simulink model "es2"  (R2024b)
settings: Solver=VariableStepAuto  StartTime=0.0  StopTime=30  RelTol=1e-3
undefined symbols (not defined in the file or in its folder): dspblkCoreblockFVToolHelper, gcbh
libraries: vrlib x1
settings Model: Creator=mattia  LastModifiedBy=elima

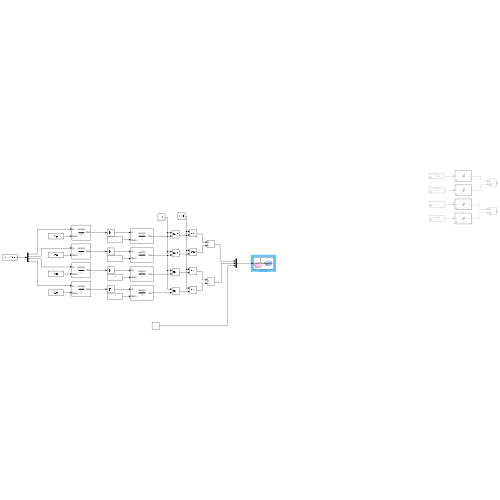
[thumbnail: Simulink's stored preview of the top-level diagram]
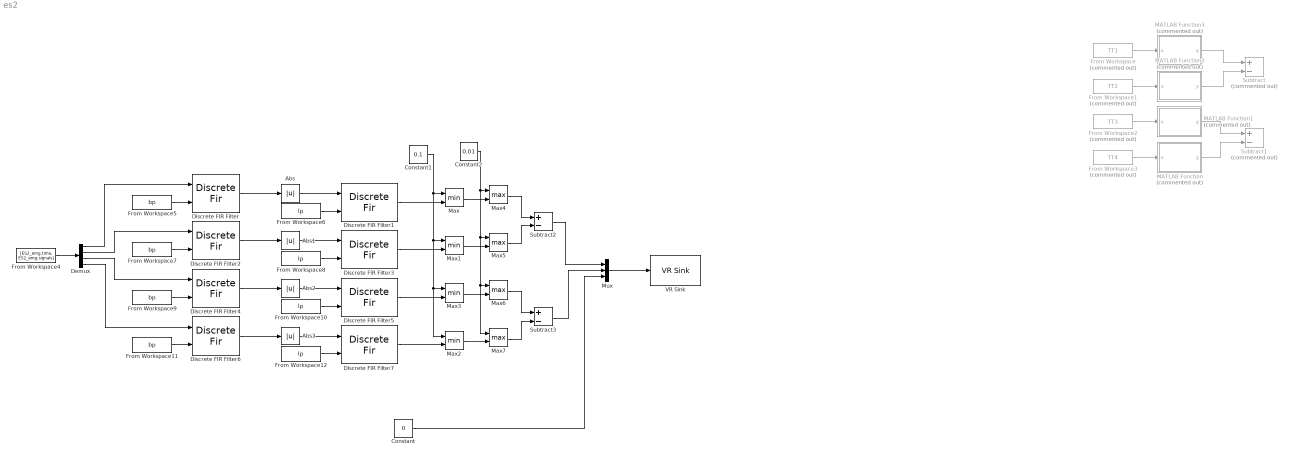
== system es2 ==
  Abs{,1..3} (4 alike) : Abs  SaturateOnIntegerOverflow=off
  Constant : Constant  Value=0
  Constant1 : Constant  Value=0.1
  Constant2 : Constant  Value=0.01
  Demux : Demux
  Discrete FIR Filter{,1..7} (8 alike) : DiscreteFir  LoadFcn=dspblkCoreblockFVToolHelper(gcbh,'load');  CoefSource=Input port
      settings: CopyFcn=dspblkCoreblockFVToolHelper(gcbh,'copy');  DeleteFcn=dspblkCoreblockFVToolHelper(gcbh,'close');  ModelCloseFcn=dspblkCoreblockFVToolHelper(gcbh,'close');  PreSaveFcn=dspblkCoreblockFVToolHelper(gcbh,'presave');  PostSaveFcn=dspblkCoreblockFVToolHelper(gcbh,'postsave');  CloseFcn=dspblkCoreblockFVToolHelper(gcbh,'close');  InputPortMap=u0,u1
  From Workspace : FromWorkspace  Commented=on  VariableName=TT1
  From Workspace1 : FromWorkspace  Commented=on  VariableName=TT2
  From Workspace{6,8,10,12} (4 alike) : FromWorkspace  VariableName=lp
  From Workspace{5,7,9,11} (4 alike) : FromWorkspace  VariableName=bp
  From Workspace2 : FromWorkspace  Commented=on  VariableName=TT3
  From Workspace3 : FromWorkspace  Commented=on  VariableName=TT4
  From Workspace4 : FromWorkspace  VariableName=[ES2_emg.time, ES2_emg.signals]  SampleTime=-1
  MATLAB Function : MATLAB Function  Commented=on  TreatAsAtomicUnit=on
  MATLAB Function1 : MATLAB Function  Commented=on  TreatAsAtomicUnit=on
  MATLAB Function2 : MATLAB Function  Commented=on  TreatAsAtomicUnit=on
  MATLAB Function3 : MATLAB Function  Commented=on  TreatAsAtomicUnit=on
  Max{,1..3} (4 alike) : MinMax  Inputs=2
  Max{4..7} (4 alike) : MinMax  Function=max  Inputs=2
  Mux : Mux  Inputs=3
  Subtract : Sum  Commented=on  Inputs=+-
  Subtract1 : Sum  Commented=on  Inputs=+-
  Subtract2 : Sum  Inputs=+-
  Subtract3 : Sum  Inputs=+-
  VR Sink : vrlib/VR Sink  InstantiateOnLoad=on  SampleTime=0.1  ViewEnable=on  RemoteChange=off  RemoteView=off  FieldsWritten=cursor.translation.3.1.1.double  WorldFileName=8_palline_color.wrl  AutoView=off  VideoDimensions=[]  AllowVariableSize=off
  wires:
  Mux/1 -> VR Sink/1
  Constant/1 -> Mux/3
  From Workspace/1 -> MATLAB Function3/1(u)
  MATLAB Function3/1(y) -> Subtract/1
  MATLAB Function2/1(y) -> Subtract/2
  MATLAB Function1/1(y) -> Subtract1/1
  MATLAB Function/1(y) -> Subtract1/2
  From Workspace1/1 -> MATLAB Function2/1(u)
  From Workspace2/1 -> MATLAB Function1/1(u)
  From Workspace3/1 -> MATLAB Function/1(u)
  From Workspace4/1 -> Demux/1
  Discrete FIR Filter/1 -> Abs/1
  Abs/1 -> Discrete FIR Filter1/1
  From Workspace5/1 -> Discrete FIR Filter/2
  From Workspace6/1 -> Discrete FIR Filter1/2
  Discrete FIR Filter2/1 -> Abs1/1
  Abs1/1 -> Discrete FIR Filter3/1
  From Workspace8/1 -> Discrete FIR Filter3/2
  From Workspace7/1 -> Discrete FIR Filter2/2
  Discrete FIR Filter4/1 -> Abs2/1
  Abs2/1 -> Discrete FIR Filter5/1
  From Workspace10/1 -> Discrete FIR Filter5/2
  From Workspace9/1 -> Discrete FIR Filter4/2
  Discrete FIR Filter6/1 -> Abs3/1
  Abs3/1 -> Discrete FIR Filter7/1
  From Workspace12/1 -> Discrete FIR Filter7/2
  From Workspace11/1 -> Discrete FIR Filter6/2
  Demux/1 -> Discrete FIR Filter/1
  Demux/2 -> Discrete FIR Filter2/1
  Demux/3 -> Discrete FIR Filter4/1
  Demux/4 -> Discrete FIR Filter6/1
  Discrete FIR Filter1/1 -> Max/2
  Discrete FIR Filter3/1 -> Max1/2
  Discrete FIR Filter5/1 -> Max3/2
  Discrete FIR Filter7/1 -> Max2/2
  Constant1/1 -> Max2/1, Max3/1, Max1/1, Max/1
  Subtract2/1 -> Mux/1
  Subtract3/1 -> Mux/2
  Max/1 -> Max4/2
  Max1/1 -> Max5/2
  Max3/1 -> Max6/2
  Max2/1 -> Max7/2
  Constant2/1 -> Max7/1, Max6/1, Max5/1, Max4/1
  Max4/1 -> Subtract2/1
  Max5/1 -> Subtract2/2
  Max6/1 -> Subtract3/1
  Max7/1 -> Subtract3/2

== matlab function es2/MATLAB Function ==
  data: u input; y output
function y = fcn(u)

val = u*0.1/0.22;

if val > 0.1 
    y = 0.1;
elseif val > 0.01
    y = val;
else 
    y = 0;
end

== matlab function es2/MATLAB Function2 ==
  data: u input; y output
function y = fcn(u)

val = u*0.1/0.008;

if val > 0.1 
    y = 0.1;
elseif val > 0.01
    y = val;
else 
    y = 0;
end

== matlab function es2/MATLAB Function3 ==
  data: u input; y output
function y = fcn(u)

val = u*0.1/0.4;

if val > 0.1 
    y = 0.1;
elseif val > 0.01
    y = val;
else 
    y = 0;
end

== matlab function es2/MATLAB Function1 ==
  data: u input; y output
function y = fcn(u)

val = u*0.1/0.2;

if val > 0.1 
    y = 0.1;
elseif val > 0.01
    y = val;
else 
    y = 0;
end
